simulink model "multi_susp_sys"  (Simulink 7.7)
settings: Solver=ode45  StartTime=0.0  StopTime=10.0  RelTol=1e-3
undefined symbols (not defined in the file): G, s, Suspension, suspension_lib
libraries: simulink x8
settings Model: Creator=jporter  LastModifiedBy=jporter

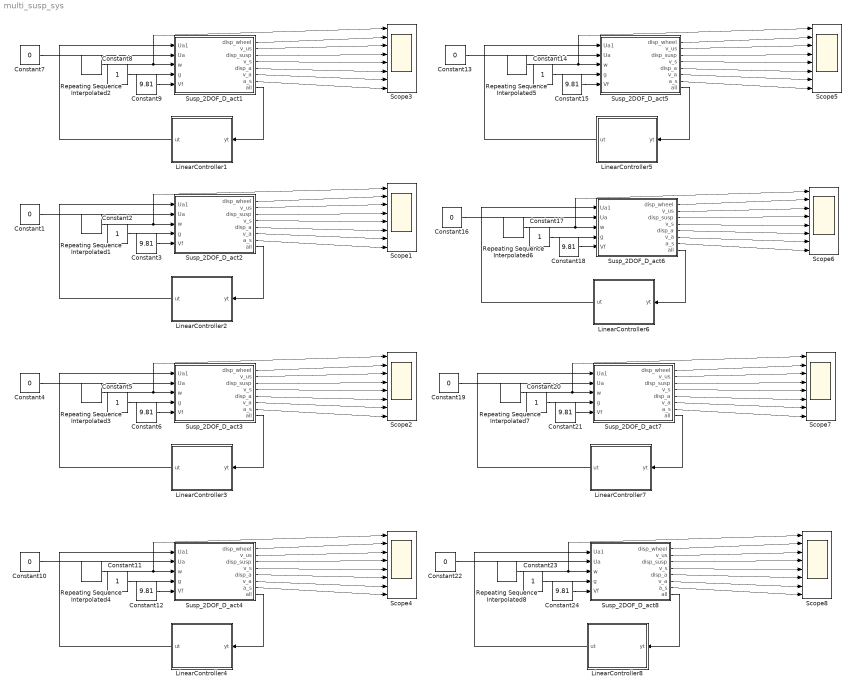
== system multi_susp_sys ==
  Constant{1,4,7,10,13,16,19,22} (8 alike) : Constant  Value=0
  Constant{2,5,8,11,14,17,20,23} (8 alike) : Constant
  Constant{3,6,9,12,15,18,21,24} (8 alike) : Constant  Value=9.81
  LinearController1 : Subsystem
  LinearController2 : Subsystem
  LinearController3 : Subsystem
  LinearController4 : Subsystem
  LinearController5 : Subsystem
  LinearController6 : Subsystem
  LinearController7 : Subsystem
  LinearController8 : Subsystem
  Repeating Sequence Interpolated{1..8} (8 alike) : simulink/Sources/Repeating Sequence Interpolated  SystemSampleTime=-1  OutValues=[0 0.5 0 -0.5 0 -0.5 0 0.5 0].'  TimeValues=[0 0.1 0.2 0.3 0.4 0.6 0.7 0.8 0.9].'  LookUpMeth=Interpolation-Use End Values  tsamp=0.01  OutMin=[]  OutMax=[]  OutDataTypeStr=double  OutputDataTypeScalingMode=double  OutDataType=fixdt(0,8)  OutScaling=2^-10
  Scope{1..8} (8 alike) : Scope  NumInputPorts=8
      Scope1 settings: YMin=-0.5~-0.5~-30~-0.9~-5~-5~-5~-5  YMax=0.5~0.5~30~0.3~5~5~5~5
      Scope2 settings: YMin=-0.5~-0.5~-30~-0.9~-5~-5~-5~-5  YMax=0.5~0.5~30~0.3~5~5~5~5  SaveName=ScopeData2
      Scope3 settings: YMin=-0.5~-0.5~-30~-0.9~-5~-5~-5~-5  YMax=0.5~0.5~30~0.3~5~5~5~5
      Scope4 settings: YMin=-0.5~-0.5~-30~-0.9~-5~-5~-5~-5  YMax=0.5~0.5~30~0.3~5~5~5~5  SaveName=ScopeData3
      Scope5 settings: YMin=-0.5~-0.5~-30~-0.9~-5~-5~-5~-5  YMax=0.5~0.5~30~0.3~5~5~5~5  SaveName=ScopeData4
      Scope6 settings: YMin=-0.5~-0.5~-30~-0.9~-5~-5~-5~-5  YMax=0.5~0.5~30~0.3~5~5~5~5  SaveName=ScopeData5
      Scope7 settings: YMin=-0.5~-0.5~-30~-0.9~-5~-5~-5~-5  YMax=0.5~0.5~30~0.3~5~5~5~5  SaveName=ScopeData6
      Scope8 settings: YMin=-0.5~-0.5~-30~-0.9~-5~-5~-5~-5  YMax=0.5~0.5~30~0.3~5~5~5~5  SaveName=ScopeData7
  Susp_2DOF_D_act1 : Subsystem  AncestorBlock=suspension_lib/Suspension:G(s)  mask{m_s=25000, k_s=60000, b_s=3500, m_us=413, k_us=65096.03, b_us=15000, m_a=0, k_a=0, b_a=0}
      mask prompts: m_s "Sprung mass (kg)"; k_s "Sprung mass spring constant (N/m)"; b_s "Sprung mass damping coefficient (N s/m)"; m_us "Unsprung mass (kg)"; k_us "Unsprung mass spring constant (N/m)"; b_us "Unsprung mass damping coefficient (N s/m)"; m_a "Damper mass (kg)"; k_a "Damper spring constant (N/m)"; b_a "Damper damping coeff (N s/m)"
      mask init:
      | w = sqrt( k_us / m_us );
      | w_us = sqrt( k_us / m_us );
      | rho = m_s / m_us;
      | rho_a = 0;
      | g = 9.81; % m/s^2 gravitational acceleration
      | 
      | % m_s == 0 and m_us == 0 are not allowed
      | % Work around possible divide by zero when m_a == 0
      | %  build A by rows
      | A = [0 1 0 0 0 0]; 
      | A = [A; -(k_us/m_us) (-b_s/m_us)+(b_us/m_us) (k_s/m_us) (b_s/m_us) 0 0]; 
      | A = [A; 0 -1 0 1 0 0]; 
      | A = [A; 0 (b_s/m_s) -(k_s/m_s) (-b_s/m_s) 0 0];
      | if ( m_a ~= 0 )
      |   w_a = sqrt( k_a / m_a );
      |   eta_a = b_a / (2 * m_a * w_a);
      |   rho_a = m_us / m_a;  
      |   A = [A; 0 -1 0 0 0 1]; 
      |   A = [A; 0 2 * eta_a * w_a 0 0 -(w_a^2) -2 * eta_a * w_a];
      | else
      |   A = [A; 0 0 0 0 0 0];
      |   A = [A; 0 0 0 0 0 0];
      | end
      | 
      | A=-A;
      | 
      | % inputs: active damper control force, 
      | %   active suspension control force,
      | %   road velocity, gravity, and sprung mass force
      | B = [0 0 -1 0 0];
      | B = [B; rho rho -(b_us/m_us) -g 0];
      | B = [B; 0 0 0 0 0];
      | B = [B; 0 -1 0 0 -1];
      | B = [B; 0 0 0 0 0];
      | B = [B; -rho * rho_a 0 0 0 0];
      | 
      | 
      | % A = [0 1 0 0 0 0]; 
      | % A = [A; -(k_us/m_us)  (-b_a/m_us) 0 0 (k_a/m_us) (b_a/m_us)]; 
      | % A = [A; 0 -1 0 1 0 0]; 
      | % A = [A; 0 0 0 0 0 0];
      | % if ( m_a ~= 0 )
      | %   w_a = sqrt( k_a / m_a );
      | %   eta_a = b_a / (2 * m_a * w_a);
      | %   rho_a = m_us / m_a;  
      | %   A = [A; 0 -1 0 0 0 1]; 
      | %   A = [A; 0 2 * eta_a * w_a 0 0 -(w_a^2) -2 * eta_a * w_a];
      | % else
      | %   A = [A; 0 0 0 0 0 0];
      | %   A = [A; 0 0 0 0 0 0];
      | % end
  Susp_2DOF_D_act2 : Subsystem  AncestorBlock=suspension_lib/Suspension:G(s)  mask{m_s=25000, k_s=60000, b_s=3500, m_us=413, k_us=65096.03, b_us=15000, m_a=0, k_a=0, b_a=0}
      mask prompts: m_s "Sprung mass (kg)"; k_s "Sprung mass spring constant (N/m)"; b_s "Sprung mass damping coefficient (N s/m)"; m_us "Unsprung mass (kg)"; k_us "Unsprung mass spring constant (N/m)"; b_us "Unsprung mass damping coefficient (N s/m)"; m_a "Damper mass (kg)"; k_a "Damper spring constant (N/m)"; b_a "Damper damping coeff (N s/m)"
      mask init: same as multi_susp_sys/Susp_2DOF_D_act1
  Susp_2DOF_D_act3 : Subsystem  AncestorBlock=suspension_lib/Suspension:G(s)  mask{m_s=25000, k_s=60000, b_s=3500, m_us=413, k_us=65096.03, b_us=15000, m_a=0, k_a=0, b_a=0}
      mask prompts: m_s "Sprung mass (kg)"; k_s "Sprung mass spring constant (N/m)"; b_s "Sprung mass damping coefficient (N s/m)"; m_us "Unsprung mass (kg)"; k_us "Unsprung mass spring constant (N/m)"; b_us "Unsprung mass damping coefficient (N s/m)"; m_a "Damper mass (kg)"; k_a "Damper spring constant (N/m)"; b_a "Damper damping coeff (N s/m)"
      mask init: same as multi_susp_sys/Susp_2DOF_D_act1
  Susp_2DOF_D_act4 : Subsystem  AncestorBlock=suspension_lib/Suspension:G(s)  mask{m_s=25000, k_s=60000, b_s=3500, m_us=413, k_us=65096.03, b_us=15000, m_a=0, k_a=0, b_a=0}
      mask prompts: m_s "Sprung mass (kg)"; k_s "Sprung mass spring constant (N/m)"; b_s "Sprung mass damping coefficient (N s/m)"; m_us "Unsprung mass (kg)"; k_us "Unsprung mass spring constant (N/m)"; b_us "Unsprung mass damping coefficient (N s/m)"; m_a "Damper mass (kg)"; k_a "Damper spring constant (N/m)"; b_a "Damper damping coeff (N s/m)"
      mask init: same as multi_susp_sys/Susp_2DOF_D_act1
  Susp_2DOF_D_act5 : Subsystem  AncestorBlock=suspension_lib/Suspension:G(s)  mask{m_s=25000, k_s=60000, b_s=3500, m_us=413, k_us=65096.03, b_us=15000, m_a=0, k_a=0, b_a=0}
      mask prompts: m_s "Sprung mass (kg)"; k_s "Sprung mass spring constant (N/m)"; b_s "Sprung mass damping coefficient (N s/m)"; m_us "Unsprung mass (kg)"; k_us "Unsprung mass spring constant (N/m)"; b_us "Unsprung mass damping coefficient (N s/m)"; m_a "Damper mass (kg)"; k_a "Damper spring constant (N/m)"; b_a "Damper damping coeff (N s/m)"
      mask init: same as multi_susp_sys/Susp_2DOF_D_act1
  Susp_2DOF_D_act6 : Subsystem  AncestorBlock=suspension_lib/Suspension:G(s)  mask{m_s=25000, k_s=60000, b_s=3500, m_us=413, k_us=65096.03, b_us=15000, m_a=0, k_a=0, b_a=0}
      mask prompts: m_s "Sprung mass (kg)"; k_s "Sprung mass spring constant (N/m)"; b_s "Sprung mass damping coefficient (N s/m)"; m_us "Unsprung mass (kg)"; k_us "Unsprung mass spring constant (N/m)"; b_us "Unsprung mass damping coefficient (N s/m)"; m_a "Damper mass (kg)"; k_a "Damper spring constant (N/m)"; b_a "Damper damping coeff (N s/m)"
      mask init: same as multi_susp_sys/Susp_2DOF_D_act1
  Susp_2DOF_D_act7 : Subsystem  AncestorBlock=suspension_lib/Suspension:G(s)  mask{m_s=25000, k_s=60000, b_s=3500, m_us=413, k_us=65096.03, b_us=15000, m_a=0, k_a=0, b_a=0}
      mask prompts: m_s "Sprung mass (kg)"; k_s "Sprung mass spring constant (N/m)"; b_s "Sprung mass damping coefficient (N s/m)"; m_us "Unsprung mass (kg)"; k_us "Unsprung mass spring constant (N/m)"; b_us "Unsprung mass damping coefficient (N s/m)"; m_a "Damper mass (kg)"; k_a "Damper spring constant (N/m)"; b_a "Damper damping coeff (N s/m)"
      mask init: same as multi_susp_sys/Susp_2DOF_D_act1
  Susp_2DOF_D_act8 : Subsystem  AncestorBlock=suspension_lib/Suspension:G(s)  mask{m_s=25000, k_s=60000, b_s=3500, m_us=413, k_us=65096.03, b_us=15000, m_a=0, k_a=0, b_a=0}
      mask prompts: m_s "Sprung mass (kg)"; k_s "Sprung mass spring constant (N/m)"; b_s "Sprung mass damping coefficient (N s/m)"; m_us "Unsprung mass (kg)"; k_us "Unsprung mass spring constant (N/m)"; b_us "Unsprung mass damping coefficient (N s/m)"; m_a "Damper mass (kg)"; k_a "Damper spring constant (N/m)"; b_a "Damper damping coeff (N s/m)"
      mask init: same as multi_susp_sys/Susp_2DOF_D_act1
  wires:
  Repeating Sequence Interpolated2/1 -> Susp_2DOF_D_act1/3(w), Scope3/1
  Susp_2DOF_D_act1/1(disp_wheel) -> Scope3/2
  Susp_2DOF_D_act1/2(v_us) -> Scope3/3
  Susp_2DOF_D_act1/3(disp_susp) -> Scope3/4
  Susp_2DOF_D_act1/4(v_s) -> Scope3/5
  Susp_2DOF_D_act1/5(disp_a) -> Scope3/6
  Susp_2DOF_D_act1/6(v_a) -> Scope3/7
  Constant7/1 -> Susp_2DOF_D_act1/2(Ua)
  Constant8/1 -> Susp_2DOF_D_act1/4(g)
  Constant9/1 -> Susp_2DOF_D_act1/5(Vf)
  Susp_2DOF_D_act1/7(a_s) -> Scope3/8
  Susp_2DOF_D_act1/8(all) -> LinearController1/1(yt)
  LinearController1/1(ut) -> Susp_2DOF_D_act1/1(Ua1)
  Repeating Sequence Interpolated1/1 -> Susp_2DOF_D_act2/3(w), Scope1/1
  Susp_2DOF_D_act2/1(disp_wheel) -> Scope1/2
  Susp_2DOF_D_act2/2(v_us) -> Scope1/3
  Susp_2DOF_D_act2/3(disp_susp) -> Scope1/4
  Susp_2DOF_D_act2/4(v_s) -> Scope1/5
  Susp_2DOF_D_act2/5(disp_a) -> Scope1/6
  Susp_2DOF_D_act2/6(v_a) -> Scope1/7
  Constant1/1 -> Susp_2DOF_D_act2/2(Ua)
  Constant2/1 -> Susp_2DOF_D_act2/4(g)
  Constant3/1 -> Susp_2DOF_D_act2/5(Vf)
  Susp_2DOF_D_act2/7(a_s) -> Scope1/8
  Susp_2DOF_D_act2/8(all) -> LinearController2/1(yt)
  LinearController2/1(ut) -> Susp_2DOF_D_act2/1(Ua1)
  Repeating Sequence Interpolated3/1 -> Susp_2DOF_D_act3/3(w), Scope2/1
  Susp_2DOF_D_act3/1(disp_wheel) -> Scope2/2
  Susp_2DOF_D_act3/2(v_us) -> Scope2/3
  Susp_2DOF_D_act3/3(disp_susp) -> Scope2/4
  Susp_2DOF_D_act3/4(v_s) -> Scope2/5
  Susp_2DOF_D_act3/5(disp_a) -> Scope2/6
  Susp_2DOF_D_act3/6(v_a) -> Scope2/7
  Constant4/1 -> Susp_2DOF_D_act3/2(Ua)
  Constant5/1 -> Susp_2DOF_D_act3/4(g)
  Constant6/1 -> Susp_2DOF_D_act3/5(Vf)
  Susp_2DOF_D_act3/7(a_s) -> Scope2/8
  Susp_2DOF_D_act3/8(all) -> LinearController3/1(yt)
  LinearController3/1(ut) -> Susp_2DOF_D_act3/1(Ua1)
  Repeating Sequence Interpolated4/1 -> Susp_2DOF_D_act4/3(w), Scope4/1
  Susp_2DOF_D_act4/1(disp_wheel) -> Scope4/2
  Susp_2DOF_D_act4/2(v_us) -> Scope4/3
  Susp_2DOF_D_act4/3(disp_susp) -> Scope4/4
  Susp_2DOF_D_act4/4(v_s) -> Scope4/5
  Susp_2DOF_D_act4/5(disp_a) -> Scope4/6
  Susp_2DOF_D_act4/6(v_a) -> Scope4/7
  Constant10/1 -> Susp_2DOF_D_act4/2(Ua)
  Constant11/1 -> Susp_2DOF_D_act4/4(g)
  Constant12/1 -> Susp_2DOF_D_act4/5(Vf)
  Susp_2DOF_D_act4/7(a_s) -> Scope4/8
  Susp_2DOF_D_act4/8(all) -> LinearController4/1(yt)
  LinearController4/1(ut) -> Susp_2DOF_D_act4/1(Ua1)
  Repeating Sequence Interpolated5/1 -> Susp_2DOF_D_act5/3(w), Scope5/1
  Susp_2DOF_D_act5/1(disp_wheel) -> Scope5/2
  Susp_2DOF_D_act5/2(v_us) -> Scope5/3
  Susp_2DOF_D_act5/3(disp_susp) -> Scope5/4
  Susp_2DOF_D_act5/4(v_s) -> Scope5/5
  Susp_2DOF_D_act5/5(disp_a) -> Scope5/6
  Susp_2DOF_D_act5/6(v_a) -> Scope5/7
  Constant13/1 -> Susp_2DOF_D_act5/2(Ua)
  Constant14/1 -> Susp_2DOF_D_act5/4(g)
  Constant15/1 -> Susp_2DOF_D_act5/5(Vf)
  Susp_2DOF_D_act5/7(a_s) -> Scope5/8
  Susp_2DOF_D_act5/8(all) -> LinearController5/1(yt)
  LinearController5/1(ut) -> Susp_2DOF_D_act5/1(Ua1)
  Repeating Sequence Interpolated6/1 -> Susp_2DOF_D_act6/3(w), Scope6/1
  Susp_2DOF_D_act6/1(disp_wheel) -> Scope6/2
  Susp_2DOF_D_act6/2(v_us) -> Scope6/3
  Susp_2DOF_D_act6/3(disp_susp) -> Scope6/4
  Susp_2DOF_D_act6/4(v_s) -> Scope6/5
  Susp_2DOF_D_act6/5(disp_a) -> Scope6/6
  Susp_2DOF_D_act6/6(v_a) -> Scope6/7
  Constant16/1 -> Susp_2DOF_D_act6/2(Ua)
  Constant17/1 -> Susp_2DOF_D_act6/4(g)
  Constant18/1 -> Susp_2DOF_D_act6/5(Vf)
  Susp_2DOF_D_act6/7(a_s) -> Scope6/8
  Susp_2DOF_D_act6/8(all) -> LinearController6/1(yt)
  LinearController6/1(ut) -> Susp_2DOF_D_act6/1(Ua1)
  Repeating Sequence Interpolated7/1 -> Susp_2DOF_D_act7/3(w), Scope7/1
  Susp_2DOF_D_act7/1(disp_wheel) -> Scope7/2
  Susp_2DOF_D_act7/2(v_us) -> Scope7/3
  Susp_2DOF_D_act7/3(disp_susp) -> Scope7/4
  Susp_2DOF_D_act7/4(v_s) -> Scope7/5
  Susp_2DOF_D_act7/5(disp_a) -> Scope7/6
  Susp_2DOF_D_act7/6(v_a) -> Scope7/7
  Constant19/1 -> Susp_2DOF_D_act7/2(Ua)
  Constant20/1 -> Susp_2DOF_D_act7/4(g)
  Constant21/1 -> Susp_2DOF_D_act7/5(Vf)
  Susp_2DOF_D_act7/7(a_s) -> Scope7/8
  Susp_2DOF_D_act7/8(all) -> LinearController7/1(yt)
  LinearController7/1(ut) -> Susp_2DOF_D_act7/1(Ua1)
  Repeating Sequence Interpolated8/1 -> Susp_2DOF_D_act8/3(w), Scope8/1
  Susp_2DOF_D_act8/1(disp_wheel) -> Scope8/2
  Susp_2DOF_D_act8/2(v_us) -> Scope8/3
  Susp_2DOF_D_act8/3(disp_susp) -> Scope8/4
  Susp_2DOF_D_act8/4(v_s) -> Scope8/5
  Susp_2DOF_D_act8/5(disp_a) -> Scope8/6
  Susp_2DOF_D_act8/6(v_a) -> Scope8/7
  Constant22/1 -> Susp_2DOF_D_act8/2(Ua)
  Constant23/1 -> Susp_2DOF_D_act8/4(g)
  Constant24/1 -> Susp_2DOF_D_act8/5(Vf)
  Susp_2DOF_D_act8/7(a_s) -> Scope8/8
  Susp_2DOF_D_act8/8(all) -> LinearController8/1(yt)
  LinearController8/1(ut) -> Susp_2DOF_D_act8/1(Ua1)

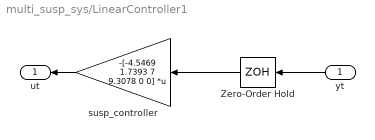
== system multi_susp_sys/LinearController1 ==
  yt : Inport
  Zero-Order Hold : ZeroOrderHold  SampleTime=0.01
  susp_controller : Gain  Gain=-[-4.5469 1.7393 7 9.3078 0 0]  Multiplication=Matrix(K*u)
  ut : Outport
  wires:
  yt/1 -> Zero-Order Hold/1
  susp_controller/1 -> ut/1
  Zero-Order Hold/1 -> susp_controller/1

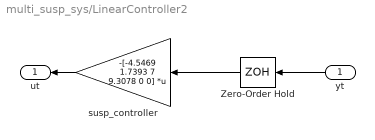
== system multi_susp_sys/LinearController2 ==
  yt : Inport
  Zero-Order Hold : ZeroOrderHold  SampleTime=0.01
  susp_controller : Gain  Gain=-[-4.5469 1.7393 7 9.3078 0 0]  Multiplication=Matrix(K*u)
  ut : Outport
  wires:
  yt/1 -> Zero-Order Hold/1
  susp_controller/1 -> ut/1
  Zero-Order Hold/1 -> susp_controller/1

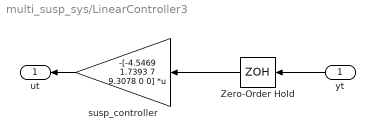
== system multi_susp_sys/LinearController3 ==
  yt : Inport
  Zero-Order Hold : ZeroOrderHold  SampleTime=0.01
  susp_controller : Gain  Gain=-[-4.5469 1.7393 7 9.3078 0 0]  Multiplication=Matrix(K*u)
  ut : Outport
  wires:
  yt/1 -> Zero-Order Hold/1
  susp_controller/1 -> ut/1
  Zero-Order Hold/1 -> susp_controller/1

== system multi_susp_sys/LinearController4 ==
  yt : Inport
  Zero-Order Hold : ZeroOrderHold  SampleTime=0.01
  susp_controller : Gain  Gain=-[-4.5469 1.7393 7 9.3078 0 0]  Multiplication=Matrix(K*u)
  ut : Outport
  wires:
  yt/1 -> Zero-Order Hold/1
  susp_controller/1 -> ut/1
  Zero-Order Hold/1 -> susp_controller/1

== system multi_susp_sys/LinearController5 ==
  yt : Inport
  Zero-Order Hold : ZeroOrderHold  SampleTime=0.01
  susp_controller : Gain  Gain=-[-4.5469 1.7393 7 9.3078 0 0]  Multiplication=Matrix(K*u)
  ut : Outport
  wires:
  yt/1 -> Zero-Order Hold/1
  susp_controller/1 -> ut/1
  Zero-Order Hold/1 -> susp_controller/1

== system multi_susp_sys/LinearController6 ==
  yt : Inport
  Zero-Order Hold : ZeroOrderHold  SampleTime=0.01
  susp_controller : Gain  Gain=-[-4.5469 1.7393 7 9.3078 0 0]  Multiplication=Matrix(K*u)
  ut : Outport
  wires:
  yt/1 -> Zero-Order Hold/1
  susp_controller/1 -> ut/1
  Zero-Order Hold/1 -> susp_controller/1

== system multi_susp_sys/LinearController7 ==
  yt : Inport
  Zero-Order Hold : ZeroOrderHold  SampleTime=0.01
  susp_controller : Gain  Gain=-[-4.5469 1.7393 7 9.3078 0 0]  Multiplication=Matrix(K*u)
  ut : Outport
  wires:
  yt/1 -> Zero-Order Hold/1
  susp_controller/1 -> ut/1
  Zero-Order Hold/1 -> susp_controller/1

== system multi_susp_sys/LinearController8 ==
  yt : Inport
  Zero-Order Hold : ZeroOrderHold  SampleTime=0.01
  susp_controller : Gain  Gain=-[-4.5469 1.7393 7 9.3078 0 0]  Multiplication=Matrix(K*u)
  ut : Outport
  wires:
  yt/1 -> Zero-Order Hold/1
  susp_controller/1 -> ut/1
  Zero-Order Hold/1 -> susp_controller/1

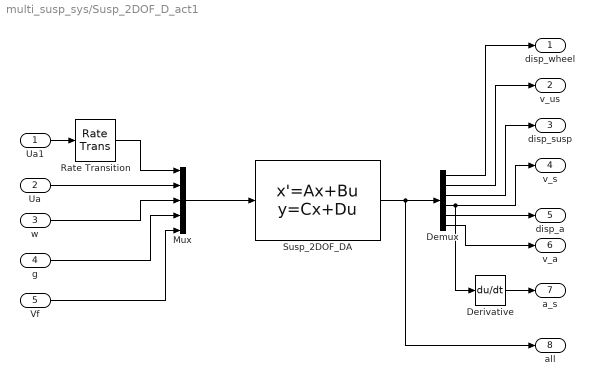
== system multi_susp_sys/Susp_2DOF_D_act1 ==
  Ua1 : Inport
  Ua : Inport  Port=2
  w : Inport  Port=3
  g : Inport  Port=4
  Vf : Inport  Port=5
  Demux : Demux  Outputs=6
  Derivative : Derivative
  Mux : Mux  Inputs=5
  Rate Transition : RateTransition
  Susp_2DOF_DA : StateSpace  A=A  B=B  C=eye(6)  D=zeros(6,5)
  disp_wheel : Outport
  v_us : Outport  Port=2
  disp_susp : Outport  Port=3
  v_s : Outport  Port=4
  disp_a : Outport  Port=5
  v_a : Outport  Port=6
  a_s : Outport  Port=7
  all : Outport  Port=8
  wires:
  Ua/1 -> Mux/2
  w/1 -> Mux/3
  Mux/1 -> Susp_2DOF_DA/1
  Susp_2DOF_DA/1 -> Demux/1, all/1
  Demux/1 -> disp_wheel/1
  Demux/2 -> v_us/1
  Demux/3 -> disp_susp/1
  Demux/4 -> v_s/1, Derivative/1
  Demux/5 -> disp_a/1
  Demux/6 -> v_a/1
  g/1 -> Mux/4
  Vf/1 -> Mux/5
  Derivative/1 -> a_s/1
  Ua1/1 -> Rate Transition/1
  Rate Transition/1 -> Mux/1

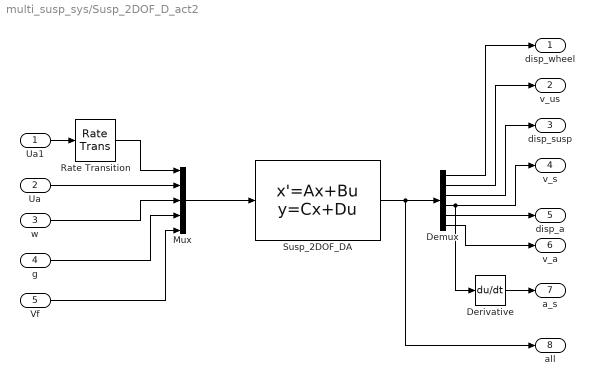
== system multi_susp_sys/Susp_2DOF_D_act2 ==
  Ua1 : Inport
  Ua : Inport  Port=2
  w : Inport  Port=3
  g : Inport  Port=4
  Vf : Inport  Port=5
  Demux : Demux  Outputs=6
  Derivative : Derivative
  Mux : Mux  Inputs=5
  Rate Transition : RateTransition
  Susp_2DOF_DA : StateSpace  A=A  B=B  C=eye(6)  D=zeros(6,5)
  disp_wheel : Outport
  v_us : Outport  Port=2
  disp_susp : Outport  Port=3
  v_s : Outport  Port=4
  disp_a : Outport  Port=5
  v_a : Outport  Port=6
  a_s : Outport  Port=7
  all : Outport  Port=8
  wires:
  Ua/1 -> Mux/2
  w/1 -> Mux/3
  Mux/1 -> Susp_2DOF_DA/1
  Susp_2DOF_DA/1 -> Demux/1, all/1
  Demux/1 -> disp_wheel/1
  Demux/2 -> v_us/1
  Demux/3 -> disp_susp/1
  Demux/4 -> v_s/1, Derivative/1
  Demux/5 -> disp_a/1
  Demux/6 -> v_a/1
  g/1 -> Mux/4
  Vf/1 -> Mux/5
  Derivative/1 -> a_s/1
  Ua1/1 -> Rate Transition/1
  Rate Transition/1 -> Mux/1

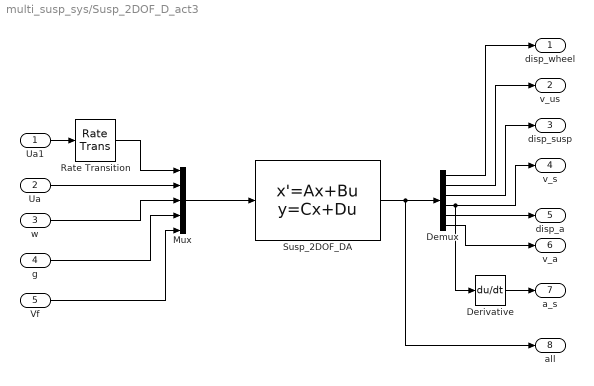
== system multi_susp_sys/Susp_2DOF_D_act3 ==
  Ua1 : Inport
  Ua : Inport  Port=2
  w : Inport  Port=3
  g : Inport  Port=4
  Vf : Inport  Port=5
  Demux : Demux  Outputs=6
  Derivative : Derivative
  Mux : Mux  Inputs=5
  Rate Transition : RateTransition
  Susp_2DOF_DA : StateSpace  A=A  B=B  C=eye(6)  D=zeros(6,5)
  disp_wheel : Outport
  v_us : Outport  Port=2
  disp_susp : Outport  Port=3
  v_s : Outport  Port=4
  disp_a : Outport  Port=5
  v_a : Outport  Port=6
  a_s : Outport  Port=7
  all : Outport  Port=8
  wires:
  Ua/1 -> Mux/2
  w/1 -> Mux/3
  Mux/1 -> Susp_2DOF_DA/1
  Susp_2DOF_DA/1 -> Demux/1, all/1
  Demux/1 -> disp_wheel/1
  Demux/2 -> v_us/1
  Demux/3 -> disp_susp/1
  Demux/4 -> v_s/1, Derivative/1
  Demux/5 -> disp_a/1
  Demux/6 -> v_a/1
  g/1 -> Mux/4
  Vf/1 -> Mux/5
  Derivative/1 -> a_s/1
  Ua1/1 -> Rate Transition/1
  Rate Transition/1 -> Mux/1

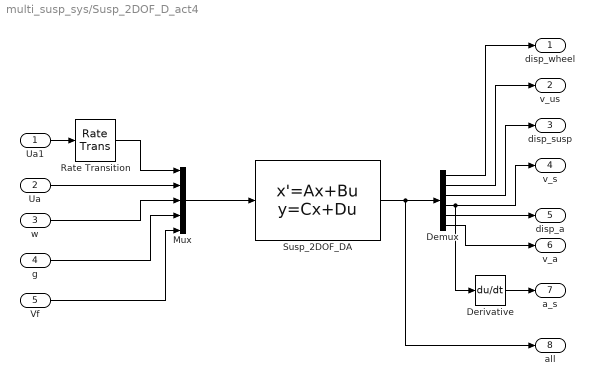
== system multi_susp_sys/Susp_2DOF_D_act4 ==
  Ua1 : Inport
  Ua : Inport  Port=2
  w : Inport  Port=3
  g : Inport  Port=4
  Vf : Inport  Port=5
  Demux : Demux  Outputs=6
  Derivative : Derivative
  Mux : Mux  Inputs=5
  Rate Transition : RateTransition
  Susp_2DOF_DA : StateSpace  A=A  B=B  C=eye(6)  D=zeros(6,5)
  disp_wheel : Outport
  v_us : Outport  Port=2
  disp_susp : Outport  Port=3
  v_s : Outport  Port=4
  disp_a : Outport  Port=5
  v_a : Outport  Port=6
  a_s : Outport  Port=7
  all : Outport  Port=8
  wires:
  Ua/1 -> Mux/2
  w/1 -> Mux/3
  Mux/1 -> Susp_2DOF_DA/1
  Susp_2DOF_DA/1 -> Demux/1, all/1
  Demux/1 -> disp_wheel/1
  Demux/2 -> v_us/1
  Demux/3 -> disp_susp/1
  Demux/4 -> v_s/1, Derivative/1
  Demux/5 -> disp_a/1
  Demux/6 -> v_a/1
  g/1 -> Mux/4
  Vf/1 -> Mux/5
  Derivative/1 -> a_s/1
  Ua1/1 -> Rate Transition/1
  Rate Transition/1 -> Mux/1

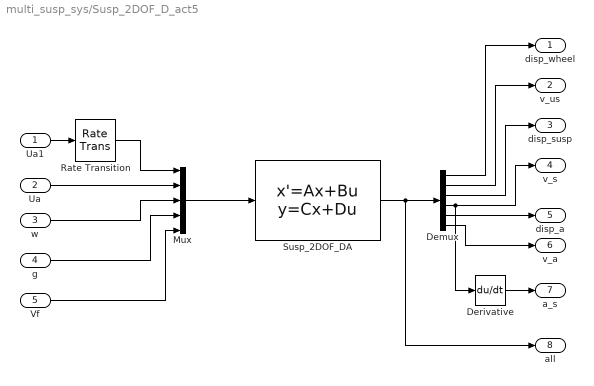
== system multi_susp_sys/Susp_2DOF_D_act5 ==
  Ua1 : Inport
  Ua : Inport  Port=2
  w : Inport  Port=3
  g : Inport  Port=4
  Vf : Inport  Port=5
  Demux : Demux  Outputs=6
  Derivative : Derivative
  Mux : Mux  Inputs=5
  Rate Transition : RateTransition
  Susp_2DOF_DA : StateSpace  A=A  B=B  C=eye(6)  D=zeros(6,5)
  disp_wheel : Outport
  v_us : Outport  Port=2
  disp_susp : Outport  Port=3
  v_s : Outport  Port=4
  disp_a : Outport  Port=5
  v_a : Outport  Port=6
  a_s : Outport  Port=7
  all : Outport  Port=8
  wires:
  Ua/1 -> Mux/2
  w/1 -> Mux/3
  Mux/1 -> Susp_2DOF_DA/1
  Susp_2DOF_DA/1 -> Demux/1, all/1
  Demux/1 -> disp_wheel/1
  Demux/2 -> v_us/1
  Demux/3 -> disp_susp/1
  Demux/4 -> v_s/1, Derivative/1
  Demux/5 -> disp_a/1
  Demux/6 -> v_a/1
  g/1 -> Mux/4
  Vf/1 -> Mux/5
  Derivative/1 -> a_s/1
  Ua1/1 -> Rate Transition/1
  Rate Transition/1 -> Mux/1

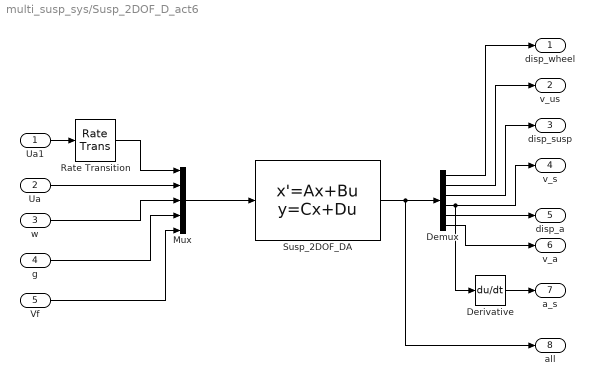
== system multi_susp_sys/Susp_2DOF_D_act6 ==
  Ua1 : Inport
  Ua : Inport  Port=2
  w : Inport  Port=3
  g : Inport  Port=4
  Vf : Inport  Port=5
  Demux : Demux  Outputs=6
  Derivative : Derivative
  Mux : Mux  Inputs=5
  Rate Transition : RateTransition
  Susp_2DOF_DA : StateSpace  A=A  B=B  C=eye(6)  D=zeros(6,5)
  disp_wheel : Outport
  v_us : Outport  Port=2
  disp_susp : Outport  Port=3
  v_s : Outport  Port=4
  disp_a : Outport  Port=5
  v_a : Outport  Port=6
  a_s : Outport  Port=7
  all : Outport  Port=8
  wires:
  Ua/1 -> Mux/2
  w/1 -> Mux/3
  Mux/1 -> Susp_2DOF_DA/1
  Susp_2DOF_DA/1 -> Demux/1, all/1
  Demux/1 -> disp_wheel/1
  Demux/2 -> v_us/1
  Demux/3 -> disp_susp/1
  Demux/4 -> v_s/1, Derivative/1
  Demux/5 -> disp_a/1
  Demux/6 -> v_a/1
  g/1 -> Mux/4
  Vf/1 -> Mux/5
  Derivative/1 -> a_s/1
  Ua1/1 -> Rate Transition/1
  Rate Transition/1 -> Mux/1

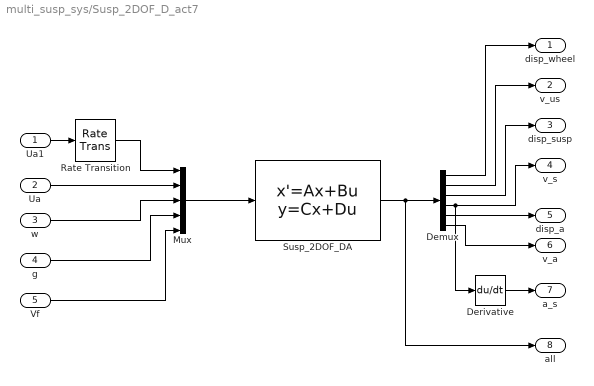
== system multi_susp_sys/Susp_2DOF_D_act7 ==
  Ua1 : Inport
  Ua : Inport  Port=2
  w : Inport  Port=3
  g : Inport  Port=4
  Vf : Inport  Port=5
  Demux : Demux  Outputs=6
  Derivative : Derivative
  Mux : Mux  Inputs=5
  Rate Transition : RateTransition
  Susp_2DOF_DA : StateSpace  A=A  B=B  C=eye(6)  D=zeros(6,5)
  disp_wheel : Outport
  v_us : Outport  Port=2
  disp_susp : Outport  Port=3
  v_s : Outport  Port=4
  disp_a : Outport  Port=5
  v_a : Outport  Port=6
  a_s : Outport  Port=7
  all : Outport  Port=8
  wires:
  Ua/1 -> Mux/2
  w/1 -> Mux/3
  Mux/1 -> Susp_2DOF_DA/1
  Susp_2DOF_DA/1 -> Demux/1, all/1
  Demux/1 -> disp_wheel/1
  Demux/2 -> v_us/1
  Demux/3 -> disp_susp/1
  Demux/4 -> v_s/1, Derivative/1
  Demux/5 -> disp_a/1
  Demux/6 -> v_a/1
  g/1 -> Mux/4
  Vf/1 -> Mux/5
  Derivative/1 -> a_s/1
  Ua1/1 -> Rate Transition/1
  Rate Transition/1 -> Mux/1

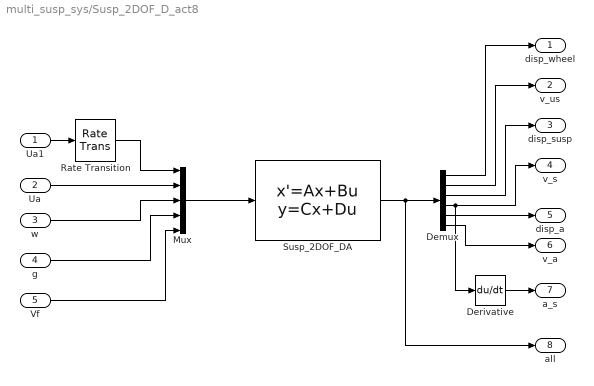
== system multi_susp_sys/Susp_2DOF_D_act8 ==
  Ua1 : Inport
  Ua : Inport  Port=2
  w : Inport  Port=3
  g : Inport  Port=4
  Vf : Inport  Port=5
  Demux : Demux  Outputs=6
  Derivative : Derivative
  Mux : Mux  Inputs=5
  Rate Transition : RateTransition
  Susp_2DOF_DA : StateSpace  A=A  B=B  C=eye(6)  D=zeros(6,5)
  disp_wheel : Outport
  v_us : Outport  Port=2
  disp_susp : Outport  Port=3
  v_s : Outport  Port=4
  disp_a : Outport  Port=5
  v_a : Outport  Port=6
  a_s : Outport  Port=7
  all : Outport  Port=8
  wires:
  Ua/1 -> Mux/2
  w/1 -> Mux/3
  Mux/1 -> Susp_2DOF_DA/1
  Susp_2DOF_DA/1 -> Demux/1, all/1
  Demux/1 -> disp_wheel/1
  Demux/2 -> v_us/1
  Demux/3 -> disp_susp/1
  Demux/4 -> v_s/1, Derivative/1
  Demux/5 -> disp_a/1
  Demux/6 -> v_a/1
  g/1 -> Mux/4
  Vf/1 -> Mux/5
  Derivative/1 -> a_s/1
  Ua1/1 -> Rate Transition/1
  Rate Transition/1 -> Mux/1
